simulink model "Beobachter"  (Simulink 8.7)
settings: Solver=VariableStepAuto  StartTime=0.0  StopTime=10.0  RelTol=1e-3
values from neighbouring files (symbols this model uses):
  L = H*P    [reglerentwurf.m]    (also in systemidentifikation.m = length(noise_in.Time); zustandsregler.m = acker(A', C', p_b)')
undefined symbols (not defined in the file or in its folder): A, B, C
settings Model: Creator=Oliver  LastModifiedBy=Oliver
settings DataIOCC: LimitDataPoints=off  SaveFormat=Dataset
settings DebuggingCC: UnderspecifiedInitializationDetection=Simplified  MergeDetectMultiDrivingBlocksExec=error
settings HardwareCC: ProdBitPerPointer=64  ProdLargestAtomicFloat=Float  ProdIntDivRoundTo=Zero  ProdEndianess=LittleEndian  ProdWordSize=64  ProdHWDeviceType=Intel->x86-64 (Windows64)
settings ModelReferenceCC: PropagateSignalLabelsOutOfModel=on
settings ConfigComp: CovModelRefEnable=off

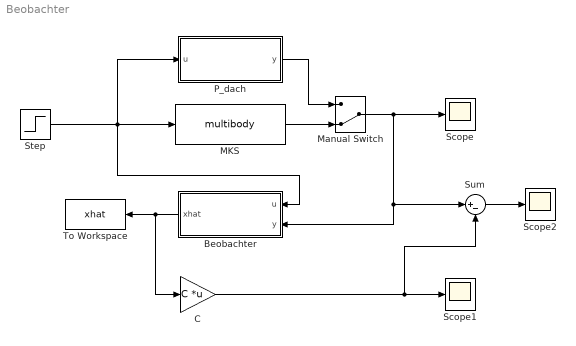
== system Beobachter ==
  Beobachter : Subsystem
  C : Gain  Gain=C  Multiplication=Matrix(K*u)
  MKS : S-Function  FunctionName=multibody  Parameters='Kiethe'  SFunctionDeploymentMode=off  EnableBusSupport=off
  Manual Switch : ManualSwitch  CurrentSetting=0
  P_dach : Subsystem
  Scope : Scope
  Scope1 : Scope
  Scope2 : Scope
  Step : Step  SampleTime=0
  Sum : Sum  Inputs=|+-
  To Workspace : ToWorkspace  VariableName=xhat  SaveFormat=Timeseries  SampleTime=-1
  wires:
  Step/1 -> P_dach/1(u), Beobachter/1(u), MKS/1
  Beobachter/1(xhat) -> C/1, To Workspace/1
  C/1 -> Sum/2, Scope1/1
  MKS/1 -> Manual Switch/2
  P_dach/1(y) -> Manual Switch/1
  Manual Switch/1 -> Scope/1, Beobachter/2(y), Sum/1
  Sum/1 -> Scope2/1

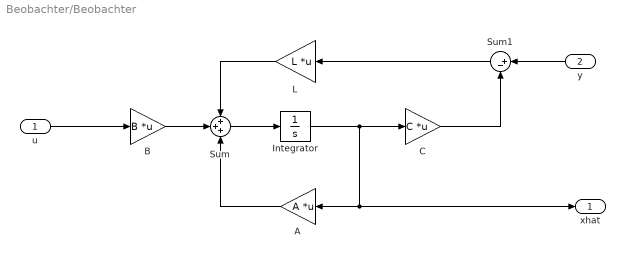
== system Beobachter/Beobachter ==
  u : Inport
  y : Inport  Port=2
  A : Gain  Gain=A  Multiplication=Matrix(K*u)
  B : Gain  Gain=B  Multiplication=Matrix(K*u)
  C : Gain  Gain=C  Multiplication=Matrix(K*u)
  Integrator : Integrator
  L : Gain  Gain=L  Multiplication=Matrix(K*u)
  Sum : Sum  Inputs=+++
  Sum1 : Sum  Inputs=|+-
  xhat : Outport
  wires:
  y/1 -> Sum1/1
  C/1 -> Sum1/2
  Sum1/1 -> L/1
  L/1 -> Sum/1
  B/1 -> Sum/2
  A/1 -> Sum/3
  Sum/1 -> Integrator/1
  Integrator/1 -> xhat/1, A/1, C/1
  u/1 -> B/1

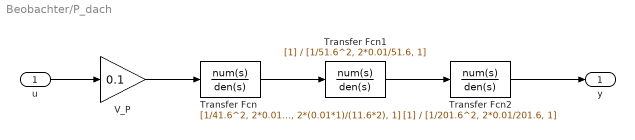
== system Beobachter/P_dach ==
  u : Inport
  Transfer Fcn : TransferFcn  Numerator=[1/41.6^2, 2*0.01/42.6, 1]  Denominator=[1/(11.6*2)^2, 2*(0.01*1)/(11.6*2), 1]
  Transfer Fcn1 : TransferFcn  Denominator=[1/51.6^2, 2*0.01/51.6, 1]
  Transfer Fcn2 : TransferFcn  Denominator=[1/201.6^2, 2*0.01/201.6, 1]
  V_P : Gain  Gain=0.1
  y : Outport
  wires:
  u/1 -> V_P/1
  V_P/1 -> Transfer Fcn/1
  Transfer Fcn/1 -> Transfer Fcn1/1
  Transfer Fcn1/1 -> Transfer Fcn2/1
  Transfer Fcn2/1 -> y/1
